simulink model "More_detailed_analysis_of_flyback"  (R2016a)
settings: Solver=VariableStepAuto  StartTime=0.0  StopTime=0.5  RelTol=1e-3
libraries: powerlib x22, powerlib_meascontrol x12
settings Model: Creator=REZA  LastModifiedBy=syf

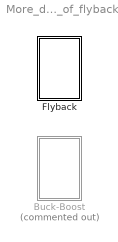
== system More_detailed_analysis_of_flyback ==
  Buck-Boost : Subsystem  Commented=on
  Flyback : Subsystem

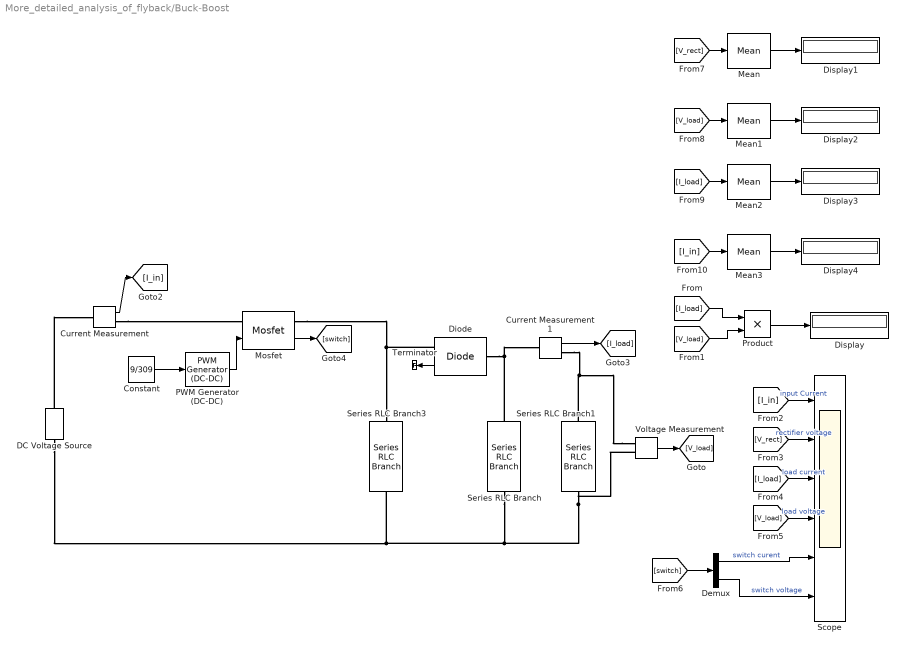
== system More_detailed_analysis_of_flyback/Buck-Boost ==
  Constant : Constant  Value=9/309
  Current Measurement : powerlib/Measurements/Current Measurement  PhasorSimulation=off  OutputType=Complex  PSBequivalent=0
  Current Measurement1 : powerlib/Measurements/Current Measurement  PhasorSimulation=off  OutputType=Complex  PSBequivalent=0
  DC Voltage Source : powerlib/Electrical Sources/DC Voltage Source  Amplitude=290  Measurements=None
  Demux : Demux  Outputs=2
  Diode : powerlib/Power Electronics/Diode  Ron=0.001  Lon=0  Vf=1.6  IC=0  UseSnubber=off  Rs=500  Cs=250e-9  Measurements=on
  Display{,1..4} (5 alike) : Display
  Mean{,1..3} (4 alike) : powerlib_meascontrol/Measurements/Mean  Freq=50  Vinit=0  Ts=0
  Mosfet : powerlib/Power Electronics/Mosfet  Ron=44e-3  Lon=0  Rd=1.2/16  Vfd=1.2  IC=0  Rs=1e5  Cs=inf  Measurements=on
  PWM Generator (DC-DC) : powerlib_meascontrol/Pulse & Signal Generators/PWM Generator (DC-DC)  Fsw=50000  Ts=0
  Product : Product
  Scope : Scope  NumInputPorts=6
  Series RLC Branch : powerlib/Elements/Series RLC Branch  LConnTagsString=__new0  RConnTagsString=__new0  BranchType=C  Resistance=1  Inductance=1e-3  SetiL0=off  InitialCurrent=0  Capacitance=4700e-6  Setx0=off  InitialVoltage=0  Measurements=None
  Series RLC Branch1 : powerlib/Elements/Series RLC Branch  LConnTagsString=__new0  RConnTagsString=__new0  BranchType=R  Resistance=8.1  Inductance=1e-3  SetiL0=off  InitialCurrent=0  Capacitance=1e-6  Setx0=off  InitialVoltage=0  Measurements=None
  Series RLC Branch3 : powerlib/Elements/Series RLC Branch  LConnTagsString=__new0  RConnTagsString=__new0  BranchType=L  Resistance=1  Inductance=92e-3  SetiL0=off  InitialCurrent=0  Capacitance=4700e-6  Setx0=off  InitialVoltage=0  Measurements=None
  Terminator : Terminator
  Voltage Measurement : powerlib/Measurements/Voltage Measurement  PhasorSimulation=off  OutputType=Complex  PSBequivalent=0
  wires:
  [V_load] -> Mean1/1
  Demux/2 -> Scope/6  "switch voltage"
  Mean1/1 -> Display2/1
  [switch] -> Demux/1
  Mean/1 -> Display1/1
  [V_rect] -> Mean/1
  Mean2/1 -> Display3/1
  Demux/1 -> Scope/5  "switch curent"
  [I_load] -> Mean2/1
  [I_in] -> Mean3/1
  Mean3/1 -> Display4/1
  Current Measurement1/1 -> [I_load]
  Constant/1 -> PWM Generator (DC-DC)/1
  [I_load] -> Scope/3  "load current"
  [I_in] -> Scope/1  "input Current"
  [I_load] -> Product/1
  Voltage Measurement/1 -> [V_load]
  Mosfet/1 -> [switch]
  PWM Generator (DC-DC)/1 -> Mosfet/1
  [V_load] -> Scope/4  "load voltage"
  Product/1 -> Display/1
  Current Measurement/1 -> [I_in]
  [V_rect] -> Scope/2  "rectifier voltage"
  [V_load] -> Product/2
  Diode/1 -> Terminator/1
  connections:
  Diode/RConn1 -- Mosfet/RConn1 -- Series RLC Branch3/LConn1
  Voltage Measurement/LConn1 -- Series RLC Branch1/RConn1 -- Current Measurement1/RConn1
  Diode/LConn1 -- Series RLC Branch/RConn1 -- Current Measurement1/LConn1
  Voltage Measurement/LConn2 -- Series RLC Branch1/LConn1 -- Series RLC Branch/LConn1 -- DC Voltage Source/LConn1 -- Series RLC Branch3/RConn1
  Current Measurement/RConn1 -- Mosfet/LConn1
  DC Voltage Source/RConn1 -- Current Measurement/LConn1

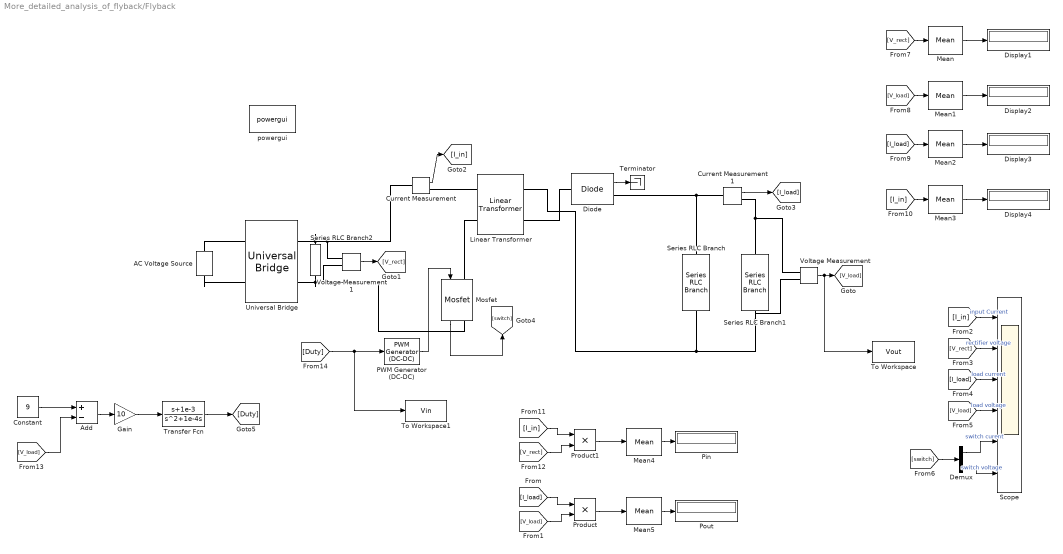
== system More_detailed_analysis_of_flyback/Flyback ==
  AC Voltage Source : powerlib/Electrical Sources/AC Voltage Source  Amplitude=230*sqrt(2)  Phase=0  Frequency=50  SampleTime=0  Measurements=None  BusType=swing  Pref=10e3  Qref=0  Qmin=-inf  Qmax=+inf
  Add : Sum  Inputs=+-
  Constant : Constant  Value=9
  Current Measurement : powerlib/Measurements/Current Measurement  PhasorSimulation=off  OutputType=Complex  PSBequivalent=0
  Current Measurement1 : powerlib/Measurements/Current Measurement  PhasorSimulation=off  OutputType=Complex  PSBequivalent=0
  Demux : Demux  Outputs=2
  Diode : powerlib/Power Electronics/Diode  Ron=0.001  Lon=0  Vf=1.6  IC=0  UseSnubber=off  Rs=500  Cs=250e-9  Measurements=on
  Display{1..4} (4 alike) : Display
  Gain : Gain  Gain=10
  Linear Transformer : powerlib/Elements/Linear Transformer  UNITS=SI  NominalPower=[ 250e6 100 ]  winding1=[190 3.2 6.8e-6]  winding2=[10 0.0142 6.8e-6]  ThreeWindings=off  winding3=[3.15e+05 0.7938 0.084225]  RmLm=[1.0805e+06 92e-3]  Measurements=None  DataType=on
  Mean{,1..5} (6 alike) : powerlib_meascontrol/Measurements/Mean  Freq=50  Vinit=0  Ts=0
  Mosfet : powerlib/Power Electronics/Mosfet  Ron=44e-3  Lon=0  Rd=1.2/16  Vfd=1.2  IC=0  Rs=1e5  Cs=inf  Measurements=on
  PWM Generator (DC-DC) : powerlib_meascontrol/Pulse & Signal Generators/PWM Generator (DC-DC)  Fsw=50000  Ts=0
  Pin : Display
  Pout : Display
  Product : Product
  Product1 : Product
  Scope : Scope  NumInputPorts=6
  Series RLC Branch : powerlib/Elements/Series RLC Branch  LConnTagsString=__new0  RConnTagsString=__new0  BranchType=C  Resistance=1  Inductance=1e-3  SetiL0=off  InitialCurrent=0  Capacitance=4700e-6  Setx0=off  InitialVoltage=0  Measurements=None
  Series RLC Branch1 : powerlib/Elements/Series RLC Branch  LConnTagsString=__new0  RConnTagsString=__new0  BranchType=R  Resistance=8.1  Inductance=1e-3  SetiL0=off  InitialCurrent=0  Capacitance=1e-6  Setx0=off  InitialVoltage=0  Measurements=None
  Series RLC Branch2 : powerlib/Elements/Series RLC Branch  LConnTagsString=__new0  RConnTagsString=__new0  BranchType=C  Resistance=1  Inductance=1e-3  SetiL0=off  InitialCurrent=0  Capacitance=47e-6  Setx0=off  InitialVoltage=0  Measurements=None
  Terminator : Terminator
  To Workspace : ToWorkspace  VariableName=Vout  SampleTime=-1
  To Workspace1 : ToWorkspace  VariableName=Vin  SampleTime=-1
  Transfer Fcn : TransferFcn  Numerator=[1 1e-3]  Denominator=[1 1e-4 0]
  Universal Bridge : powerlib/Power Electronics/Universal Bridge  Arms=2  SnubberResistance=1e5  SnubberCapacitance=inf  Device=Diodes  Ron=1e-3  Lon=0  ForwardVoltages="[  0  0  ]"  ForwardVoltage=0  GTOparameters=[ 10e-6 , 20e-6 ]  IGBTparameters=[ 1e-6 , 2e-6 ]  Measurements=None  Measurements_2=None  converterType=Rectifier
  Voltage Measurement : powerlib/Measurements/Voltage Measurement  PhasorSimulation=off  OutputType=Complex  PSBequivalent=0
  Voltage Measurement1 : powerlib/Measurements/Voltage Measurement  PhasorSimulation=off  OutputType=Complex  PSBequivalent=0
  powergui : powerlib/powergui  Priority=1  SimulationMode=Continuous  SolverType=Tustin/Backward Euler (TBE)  SampleTime=50e-6  frequency=60  SPID=on  DisableSnubberDevices=off  DisableRonSwitches=off  DisableVfSwitches=off  SwTol=0  DisplayEquations=off  Interpol=off  ExternalGateDelay=off  methode=off  Ts=10  FunctionMessages=off  echomessages=off  HookPort=off  EnableUseOfTLC=off  x0status=blocks  frequencyindice=0  Pbase=100e6  ErrMax=1e-4  Iterations=50  UnitsV=kV  UnitsW=MW  buscounter=0  RestoreLinks=warning  ResistiveCurrentMeasurement=off  Frange=[0:2:500]  Ylog=off  Xlog=on  ShowGrid=off  save=off  variable=ZData  structure=0  ZoomFFT=off  StartTime=0.0  cycles=1  DisplayStyle=1  fundamental=60  FreqAxis=off  MaxFrequency=1000  frequencyindicesteady=1  RmsSteady=1  display=off
  wires:
  Diode/1 -> Terminator/1
  [V_load] -> Product/2
  [V_rect] -> Scope/2  "rectifier voltage"
  Current Measurement/1 -> [I_in]
  Product/1 -> Mean5/1
  [V_load] -> Scope/4  "load voltage"
  PWM Generator (DC-DC)/1 -> Mosfet/1
  Mosfet/1 -> [switch]
  Voltage Measurement/1 -> To Workspace/1, [V_load]
  [I_load] -> Product/1
  [I_in] -> Scope/1  "input Current"
  [I_load] -> Scope/3  "load current"
  [Duty] -> PWM Generator (DC-DC)/1, To Workspace1/1
  Voltage Measurement1/1 -> [V_rect]
  Current Measurement1/1 -> [I_load]
  Mean3/1 -> Display4/1
  [I_in] -> Mean3/1
  [I_load] -> Mean2/1
  Demux/1 -> Scope/5  "switch curent"
  Mean2/1 -> Display3/1
  [V_rect] -> Mean/1
  Mean/1 -> Display1/1
  [switch] -> Demux/1
  Mean1/1 -> Display2/1
  Demux/2 -> Scope/6  "switch voltage"
  [V_load] -> Mean1/1
  [V_rect] -> Product1/2
  Product1/1 -> Mean4/1
  [I_in] -> Product1/1
  Mean4/1 -> Pin/1
  Mean5/1 -> Pout/1
  Gain/1 -> Transfer Fcn/1
  Add/1 -> Gain/1
  Constant/1 -> Add/1
  [V_load] -> Add/2
  Transfer Fcn/1 -> [Duty]
  connections:
  Linear Transformer/LConn1 -- Current Measurement/RConn1
  AC Voltage Source/LConn1 -- Universal Bridge/LConn2
  Series RLC Branch1/RConn1 -- Linear Transformer/RConn1 -- Series RLC Branch/RConn1 -- Voltage Measurement/LConn2
  Universal Bridge/RConn1 -- Series RLC Branch2/LConn1 -- Voltage Measurement1/LConn1 -- Current Measurement/LConn1
  AC Voltage Source/RConn1 -- Universal Bridge/LConn1
  Series RLC Branch/LConn1 -- Current Measurement1/LConn1 -- Diode/RConn1
  Series RLC Branch1/LConn1 -- Current Measurement1/RConn1 -- Voltage Measurement/LConn1
  Universal Bridge/RConn2 -- Series RLC Branch2/RConn1 -- Mosfet/RConn1 -- Voltage Measurement1/LConn2
  Linear Transformer/RConn2 -- Diode/LConn1
  Mosfet/LConn1 -- Linear Transformer/LConn2
